simulink model "Multirotor_Mixer"  (R2023b)
settings: Solver=VariableStepAuto  StartTime=0.0  StopTime=10.0  RelTol=1e-3
undefined symbols (not defined in the file): allocation_matrix, omega_nom, thrust_scale, yaw_scale
libraries: simulink x1
settings Model: Creator=Saif Mohamed  LastModifiedBy=saifg

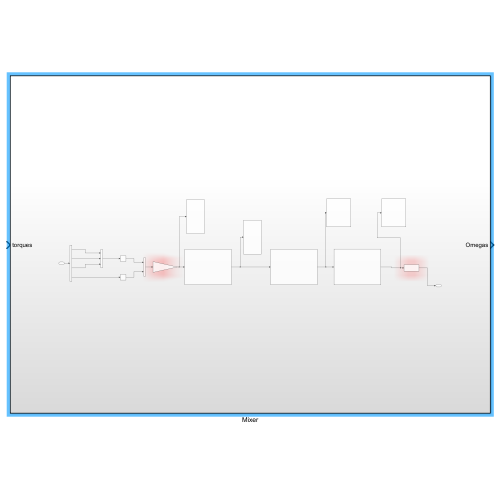
[thumbnail: Simulink's stored preview of the top-level diagram]
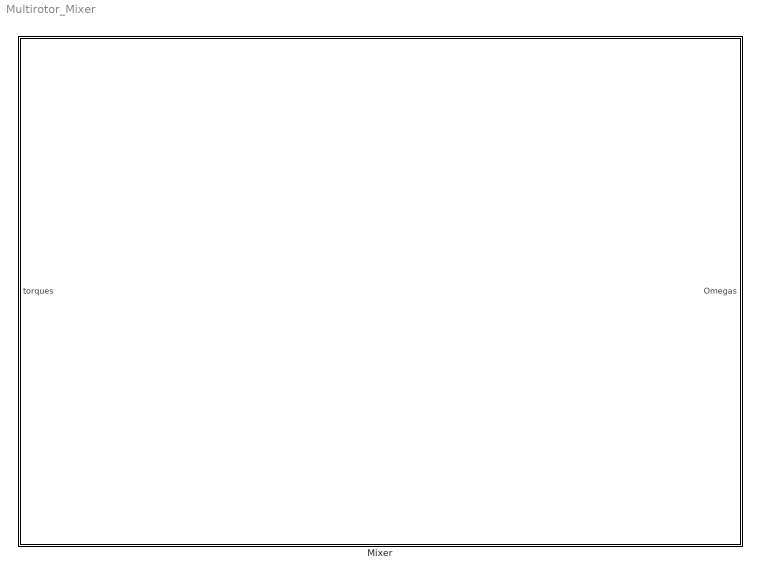
== system Multirotor_Mixer ==
  Mixer : Subsystem

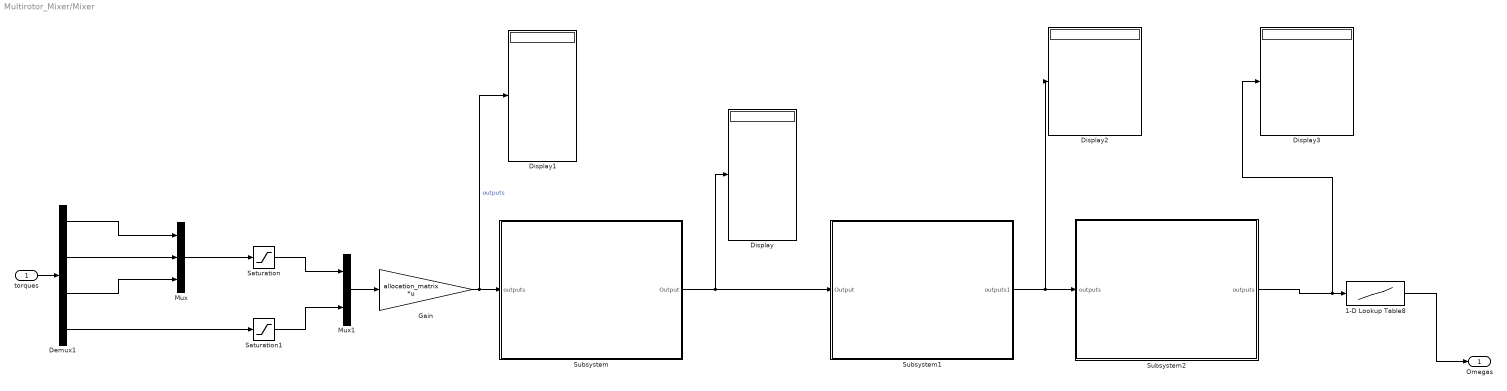
== system Multirotor_Mixer/Mixer ==
  torques : Inport
  1-D Lookup Table8 : Lookup_n-D  NumberOfTableDimensions=1  BreakpointsForDimension1=[-1 0 1]  Table="[omega_nom/2     omega_nom     sqrt(1.7)*omega_nom]"  InterpMethod=Akima spline  InternalRulePriority=Speed  RndMeth=Simplest
  Demux1 : Demux
  Display{,1..3} (4 alike) : Display
  Gain : Gain  Gain=allocation_matrix  Multiplication=Matrix(K*u)
  Mux : Mux  Inputs=3
  Mux1 : Mux  Inputs=2
  Saturation : Saturate  UpperLimit=1  LowerLimit=-1
  Saturation1 : Saturate  UpperLimit=1  LowerLimit=0
  Subsystem : Subsystem
  Subsystem1 : Subsystem
  Subsystem2 : Subsystem
  Omegas : Outport
  wires:
  torques/1 -> Demux1/1
  Demux1/1 -> Mux/1
  Demux1/2 -> Mux/2
  Demux1/3 -> Mux/3
  Mux/1 -> Saturation/1
  Demux1/4 -> Saturation1/1
  Saturation/1 -> Mux1/1
  Saturation1/1 -> Mux1/2
  Mux1/1 -> Gain/1
  Gain/1 -> Display1/1, Subsystem/1(outputs)  "outputs"
  Subsystem1/1(outputs1) -> Display2/1, Subsystem2/1("outputs ")
  Subsystem2/1(outputs) -> Display3/1, 1-D Lookup Table8/1
  Subsystem/1(Output) -> Subsystem1/1(Output), Display/1
  1-D Lookup Table8/1 -> Omegas/1

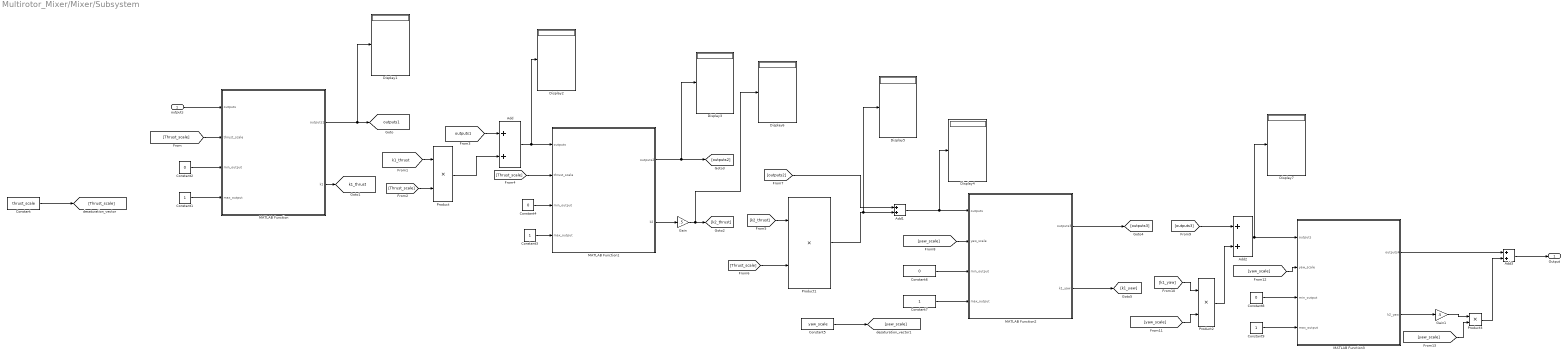
== system Multirotor_Mixer/Mixer/Subsystem ==
  outputs : Inport
  Add{,1..3} (4 alike) : Sum
  Constant : Constant  Value=thrust_scale
  Constant{1,3,7,9} (4 alike) : Constant
  Constant{2,4,6,8} (4 alike) : Constant  Value=0
  Constant5 : Constant  Value=yaw_scale
  Display{1..7} (7 alike) : Display
  Gain : Gain  Gain=.5
  Gain1 : Gain  Gain=.5
  MATLAB Function : MATLAB Function  TreatAsAtomicUnit=on
  MATLAB Function1 : MATLAB Function  TreatAsAtomicUnit=on
  MATLAB Function2 : MATLAB Function  TreatAsAtomicUnit=on
  MATLAB Function3 : MATLAB Function  TreatAsAtomicUnit=on
  Product{,1..3} (4 alike) : Product
  Output : Outport
  tag scope: k1_thrust=global, outputs1=global
  wires:
  outputs/1 -> MATLAB Function/1(outputs)
  Constant1/1 -> MATLAB Function/4(max_output)
  Constant2/1 -> MATLAB Function/3(min_output)
  Constant/1 -> [Thrust_scale]
  [Thrust_scale] -> MATLAB Function/2(thrust_scale)
  MATLAB Function/2(k1) -> [k1_thrust]
  [k1_thrust] -> Product/1
  [Thrust_scale] -> Product/2
  Product/1 -> Add/2
  [outputs1] -> Add/1
  Add/1 -> Display2/1, MATLAB Function1/1(outputs)
  [Thrust_scale] -> MATLAB Function1/2(thrust_scale)
  Constant3/1 -> MATLAB Function1/4(max_output)
  Constant4/1 -> MATLAB Function1/3(min_output)
  MATLAB Function1/2(k2) -> Gain/1
  Gain/1 -> Display6/1, [k2_thrust]
  MATLAB Function1/1(outputs2) -> Display3/1, [outputs2]
  [k2_thrust] -> Product1/1
  [Thrust_scale] -> Product1/2
  Product1/1 -> Display5/1, Add1/2
  [outputs2] -> Add1/1
  Constant5/1 -> [yaw_scale]
  [yaw_scale] -> MATLAB Function2/2(yaw_scale)
  Constant6/1 -> MATLAB Function2/3(min_output)
  Constant7/1 -> MATLAB Function2/4(max_output)
  MATLAB Function2/1(outputs3) -> [outputs3]
  MATLAB Function2/2(k1_yaw) -> [k1_yaw]
  [outputs3] -> Add2/1
  [k1_yaw] -> Product2/1
  [yaw_scale] -> Product2/2
  Product2/1 -> Add2/2
  [yaw_scale] -> MATLAB Function3/2(yaw_scale)
  Constant8/1 -> MATLAB Function3/3(min_output)
  Constant9/1 -> MATLAB Function3/4(max_output)
  MATLAB Function3/1(outputs4) -> Add3/1
  MATLAB Function3/2(k2_yaw) -> Gain1/1
  Gain1/1 -> Product3/1
  [yaw_scale] -> Product3/2
  Product3/1 -> Add3/2
  Add3/1 -> Output/1
  MATLAB Function/1(outputs1) -> Display1/1, [outputs1]
  Add1/1 -> Display4/1, MATLAB Function2/1(outputs)
  Add2/1 -> Display7/1, MATLAB Function3/1(outputs)

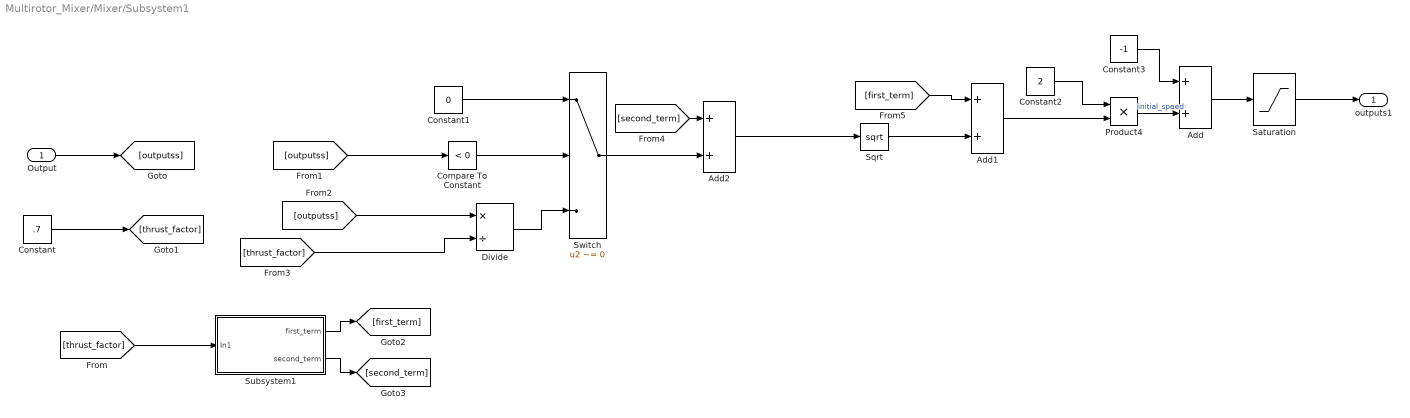
== system Multirotor_Mixer/Mixer/Subsystem1 ==
  Output : Inport
  Add : Sum
  Add1 : Sum
  Add2 : Sum
  Compare To Constant : simulink/Logic and Bit Operations/Compare To Constant  relop=<  const=0  OutDataTypeStr=boolean
  Constant : Constant  Value=.7
  Constant1 : Constant  Value=0
  Constant2 : Constant  Value=2
  Constant3 : Constant  Value=-1
  Divide : Product  Inputs=*/
  Product4 : Product
  Saturation : Saturate  UpperLimit=1  LowerLimit=-1
  Sqrt : Sqrt
  Subsystem1 : Subsystem
  Switch : Switch  Criteria=u2 ~= 0  SaturateOnIntegerOverflow=off  InputSameDT=off
  outputs1 : Outport
  wires:
  Output/1 -> [outputss]
  Constant/1 -> [thrust_factor]
  [thrust_factor] -> Subsystem1/1(In1)
  Subsystem1/1(first_term) -> [first_term]
  Subsystem1/2(second_term) -> [second_term]
  [outputss] -> Compare To Constant/1
  Compare To Constant/1 -> Switch/2
  Constant1/1 -> Switch/1
  Divide/1 -> Switch/3
  Switch/1 -> Add2/2
  [second_term] -> Add2/1
  Add2/1 -> Sqrt/1
  Sqrt/1 -> Add1/2
  [first_term] -> Add1/1
  Add1/1 -> Product4/2
  Constant2/1 -> Product4/1
  Product4/1 -> Add/2  "initial_speed"
  Constant3/1 -> Add/1
  Add/1 -> Saturation/1
  Saturation/1 -> outputs1/1
  [outputss] -> Divide/1
  [thrust_factor] -> Divide/2

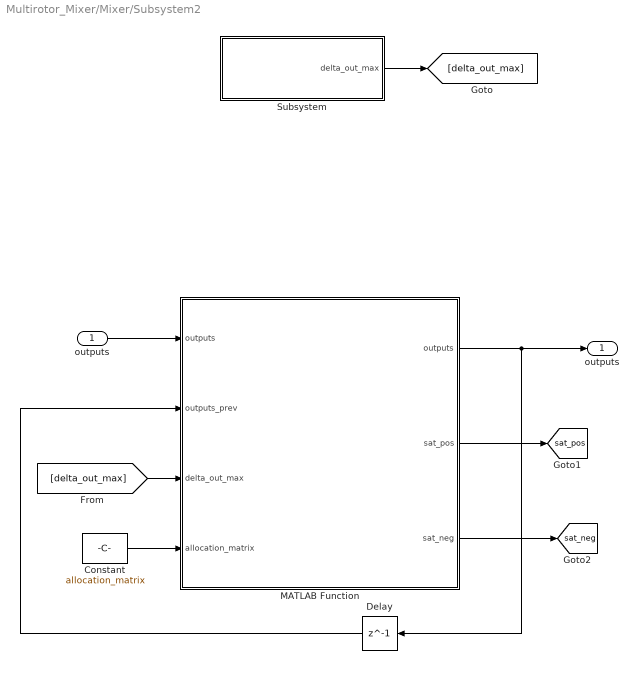
== system Multirotor_Mixer/Mixer/Subsystem2 ==
  "outputs " : Inport
  Constant : Constant  Value=allocation_matrix
  Delay : Delay  DelayLength=1
  MATLAB Function : MATLAB Function  TreatAsAtomicUnit=on
  Subsystem : Subsystem
  outputs : Outport
  tag scope: sat_neg=global, sat_pos=global
  wires:
  Subsystem/1(delta_out_max) -> [delta_out_max]
  MATLAB Function/1(outputs) -> Delay/1, outputs/1
  Delay/1 -> MATLAB Function/2(outputs_prev)
  "outputs "/1 -> MATLAB Function/1("outputs ")
  [delta_out_max] -> MATLAB Function/3(delta_out_max)
  Constant/1 -> MATLAB Function/4(allocation_matrix)
  MATLAB Function/2(sat_pos) -> [sat_pos]
  MATLAB Function/3(sat_neg) -> [sat_neg]

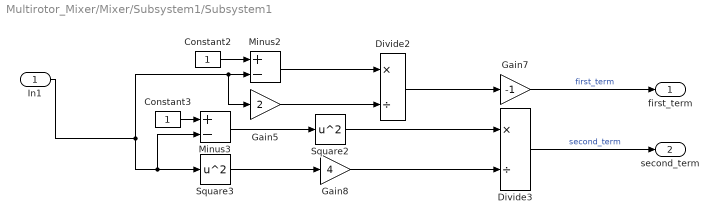
== system Multirotor_Mixer/Mixer/Subsystem1/Subsystem1 ==
  In1 : Inport
  Constant2 : Constant
  Constant3 : Constant
  Divide2 : Product  Inputs=*/
  Divide3 : Product  Inputs=*/
  Gain5 : Gain  Gain=2
  Gain7 : Gain  Gain=-1
  Gain8 : Gain  Gain=4
  Minus2 : Sum  Inputs=+-
  Minus3 : Sum  Inputs=+-
  Square2 : Math  Operator=square
  Square3 : Math  Operator=square
  first_term : Outport
  second_term : Outport  Port=2
  wires:
  Gain7/1 -> first_term/1  "first_term"
  Square3/1 -> Gain8/1
  Gain5/1 -> Divide2/2
  Gain8/1 -> Divide3/2
  Divide2/1 -> Gain7/1
  Square2/1 -> Divide3/1
  Divide3/1 -> second_term/1  "second_term"
  Minus2/1 -> Divide2/1
  Constant3/1 -> Minus3/1
  In1/1 -> Minus2/2, Gain5/1, Minus3/2, Square3/1
  Minus3/1 -> Square2/1
  Constant2/1 -> Minus2/1

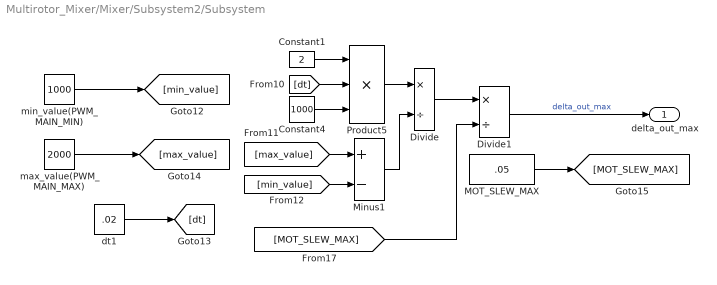
== system Multirotor_Mixer/Mixer/Subsystem2/Subsystem ==
  Constant1 : Constant  Value=2
  Constant4 : Constant  Value=1000
  Divide : Product  Inputs=*/
  Divide1 : Product  Inputs=*/
  MOT_SLEW_MAX : Constant  Value=.05
  Minus1 : Sum  Inputs=+-
  Product5 : Product  Inputs=3
  dt1 : Constant  Value=.02
  max_value(PWM_MAIN_MAX) : Constant  Value=2000
  min_value(PWM_MAIN_MIN) : Constant  Value=1000
  delta_out_max : Outport
  wires:
  max_value(PWM_MAIN_MAX)/1 -> [max_value]
  [dt] -> Product5/2
  Constant4/1 -> Product5/3
  MOT_SLEW_MAX/1 -> [MOT_SLEW_MAX]
  Divide1/1 -> delta_out_max/1  "delta_out_max"
  dt1/1 -> [dt]
  Constant1/1 -> Product5/1
  min_value(PWM_MAIN_MIN)/1 -> [min_value]
  [max_value] -> Minus1/1
  Divide/1 -> Divide1/1
  [min_value] -> Minus1/2
  Minus1/1 -> Divide/2
  Product5/1 -> Divide/1
  [MOT_SLEW_MAX] -> Divide1/2

== matlab function Multirotor_Mixer/Mixer/Subsystem/MATLAB Function1 ==
  data: outputs input; outputs2 output; thrust_scale input; min_output input; max_output input; k2 output
function [outputs2,k2] = fcn(outputs,thrust_scale,min_output,max_output)
k_min = 0;
k_max = 0;


for  i = 1:8 
    if(outputs(i)< min_output)
       k = (min_output - outputs(i)) / thrust_scale(i);

            if (k < k_min)
                 k_min = k; 
            end
            
            if (k > k_max)
                 k_max = k; 
            end
            
    end
    
    if (outputs(i)> max_output)
        
            k = (max_output - outputs(i)) / thrust_scale(i);

            if (k < k_min)
                 k_min = k; 
            end
            
            if (k > k_max)
                 k_max = k; 
            end
            
    end
end
k2 = k_min+k_max;


outputs2=outputs;

== matlab function Multirotor_Mixer/Mixer/Subsystem/MATLAB Function ==
  data: outputs input; outputs1 output; thrust_scale input; min_output input; max_output input; k1 output
function [outputs1,k1] = fcn(outputs,thrust_scale,min_output,max_output)
k_min = 0;
k_max = 0;


motor_neg = zeros(8,1);
motor_pos = zeros(8,1);

for  i = 1:8 
    if(outputs(i)< min_output)
       k = (min_output - outputs(i)) / thrust_scale(i);

            if (k < k_min)
                 k_min = k; 
            end
            
            if (k > k_max)
                 k_max = k; 
            end
            
			motor_neg(i) = 1;
    end
    
    if (outputs(i)> max_output)
        
            k = (max_output - outputs(i)) / thrust_scale(i);

            if (k < k_min)
                 k_min = k; 
            end
            
            if (k > k_max)
                 k_max = k; 
            end
            
			motor_pos(i) = 1;
    end
end
k1 = k_min+k_max;











outputs1=outputs;

== matlab function Multirotor_Mixer/Mixer/Subsystem/MATLAB Function2 ==
  data: outputs input; outputs3 output; yaw_scale input; min_output input; max_output input; k1_yaw output
function [outputs3,k1_yaw] = fcn(outputs,yaw_scale,min_output,max_output)
k_min = 0;
k_max = 0;


for  i = 1:8 
    if(outputs(i)< min_output)
       k = (min_output - outputs(i)) / yaw_scale(i);

            if (k < k_min)
                 k_min = k; 
            end
            
            if (k > k_max)
                 k_max = k; 
            end
            
    end
    
    if (outputs(i)> max_output)
        
            k = (max_output - outputs(i)) / yaw_scale(i);

            if (k < k_min)
                 k_min = k; 
            end
            
            if (k > k_max)
                 k_max = k; 
            end
            
    end
end
k1_yaw = k_min+k_max;

outputs3=outputs;

== matlab function Multirotor_Mixer/Mixer/Subsystem/MATLAB Function3 ==
  data: outputs input; outputs4 output; yaw_scale input; min_output input; max_output input; k2_yaw output
function [outputs4,k2_yaw] = fcn(outputs,yaw_scale,min_output,max_output)
k_min = 0;
k_max = 0;

for  i = 1:8 
    if(outputs(i)< min_output)
       k = (min_output - outputs(i)) / yaw_scale(i);

            if (k < k_min)
                 k_min = k; 
            end
            
            if (k > k_max)
                 k_max = k; 
            end
            
    end
    
    if (outputs(i)> max_output)
        
            k = (max_output - outputs(i)) / yaw_scale(i);

            if (k < k_min)
                 k_min = k; 
            end
            
            if (k > k_max)
                 k_max = k; 
            end
            
    end
end
k2_yaw = k_min+k_max;


outputs4=outputs;

== matlab function Multirotor_Mixer/Mixer/Subsystem2/MATLAB Function ==
  data: outputs input; outputs output; outputs_prev input; delta_out_max input; allocation_matrix input; sat_pos output; sat_neg output
function [outputs,sat_pos,sat_neg] = fcn(outputs,outputs_prev,delta_out_max,allocation_matrix)


roll_pos = 0;
roll_neg = 0;
pitch_pos = 0;
pitch_neg = 0;
yaw_pos = 0;
yaw_neg = 0;
thrust_pos = 0;
thrust_neg = 0;

for i=1:8
    clipping_high = 0;
    clipping_low_roll_pitch = 0;
    clipping_low_yaw = 0;
    

    
    if (delta_out_max > 0)
        delta_out = outputs(i) - outputs_prev(i);
        
        if (delta_out > delta_out_max)
            outputs(i) = outputs_prev(i) + delta_out_max;
            clipping_high = 1;
            
        elseif (delta_out < -delta_out_max)
            outputs(i) = outputs_prev(i) - delta_out_max;
            clipping_low_roll_pitch = 1;
            clipping_low_yaw = 1;
        end
    end
    
    outputs_prev(i) = outputs(i);
    
    if (clipping_high == 1)
        if (allocation_matrix(i,1) > 0)
            roll_pos = 1;
            
        elseif (allocation_matrix(i,1)< 0)
            roll_neg = 1;
        end
        
        if (allocation_matrix(i,2) > 0)
            pitch_pos = 1;
            
        elseif (allocation_matrix(i,2) < 0)
            pitch_neg = 1;
        end
        
        if (allocation_matrix(i,3) > 0)
            yaw_pos = 1;
            
        elseif (allocation_matrix(i,3) < 0)
            yaw_neg = 1;
        end
        
        % 		// A positive change in thrust will increase saturation
        thrust_pos = 1;
    end
    
    % 	// The motor is saturated at the lower limit
    % 	// check which control axes and which directions are contributing
    if (clipping_low_roll_pitch == 1)
        % 		// check if the roll input is saturating
        if (allocation_matrix(i,1) > 0)
            % 			// A negative change in roll will increase saturation
            roll_neg = 1;
            
        elseif (allocation_matrix(i,1) < 0)
            roll_pos = 1;
        end
        
        if (allocation_matrix(i,2) > 0)
            pitch_neg = 1;
            
        elseif (allocation_matrix(i,2) < 0)
            pitch_pos = 1;
        end
        
        thrust_neg = 1;
    end
    
    if (clipping_low_yaw == 1)
        if (allocation_matrix(i,3) > 0)
            yaw_neg = 1;
            
        elseif (allocation_matrix(i,3) < 0)
            yaw_pos = 1;
        end
    end
    
    
end
sat_pos = [roll_pos,pitch_pos,yaw_pos];
sat_neg = [roll_neg,pitch_neg,yaw_neg];
